simulink model "SIMULINK_anti-windup_anti-saturation"  (R2024b)
settings: Solver=ode45  StartTime=0.0  StopTime=1000  RelTol=1e-7  EnableMultiTasking=on
undefined symbols (not defined in the file): procede
settings Model: Creator=LiberT  LastModifiedBy=lordo
settings SolverCC: AlgebraicLoopSolver=TrustRegion
settings DataIOCC: LimitDataPoints=on  SaveFormat=Array  SignalLoggingSaveFormat=ModelDataLogs  ReturnWorkspaceOutputs=off
settings OptimizationCC: BlockReduction=off  BooleanDataType=off  ExpressionDepthLimit=2147483647  InitFltsAndDblsToZero=on  LifeSpan=inf
settings DebuggingCC: SaveWithParameterizedLinksMsg=none  UnderspecifiedInitializationDetection=Classic  MergeDetectMultiDrivingBlocksExec=none  SignalResolutionControl=TryResolveAllWithWarning  MultiTaskDSMMsg=warning  MultiTaskCondExecSysMsg=none  FcnCallInpInsideContextMsg=warning  UnconnectedInputMsg=warning  UnconnectedOutputMsg=warning  UnconnectedLineMsg=warning  StateNameClashWarn=warning  SFUnexpectedBacktrackingDiag=warning  SFNoUnconditionalDefaultTransitionDiag=warning  SFExecutionAtInitializationDiag=none  ArithmeticOperatorsInVariantConditions=warning
settings HardwareCC: ProdBitPerPointer=32  ProdBitPerSizeT=32  ProdBitPerPtrDiffT=32  ProdLargestAtomicFloat=None  ProdIntDivRoundTo=Undefined  ProdEndianess=Unspecified  ProdWordSize=32  ProdHWDeviceType=32-bit Generic  TargetUnknown=on
settings ModelReferenceCC: EnableRefExpFcnMdlSchedulingChecks=on  PropagateSignalLabelsOutOfModel=off
settings SFSimCC: SimUseLocalCustomCode=off  CustomCodeUndefinedFunction=UseInterfaceOnly
settings RTWCC: RTWUseLocalCustomCode=off  GPUComputeCapability=3.5
settings CodeAppCC: StateflowObjectComments=on
settings GRTTargetCC: TargetFcnLib=ansi_tfl_tmw.mat  TargetLangStandard=C89/C90 (ANSI)  ModelReferenceCompliant=off  CompOptLevelCompliant=off  CombineOutputUpdateFcns=off  MatFileLogging=off  GRTInterface=on
settings ConfigComp: CovMetricSettings=dw  CovSaveCumulativeToWorkspaceVar=on  CovSaveSingleToWorkspaceVar=on  CovExternalEMLEnable=off

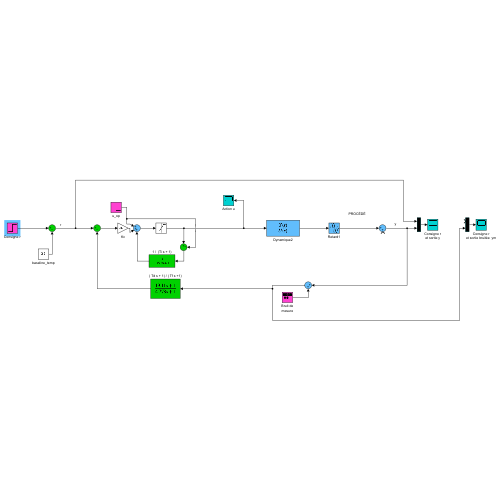
[thumbnail: Simulink's stored preview of the top-level diagram]
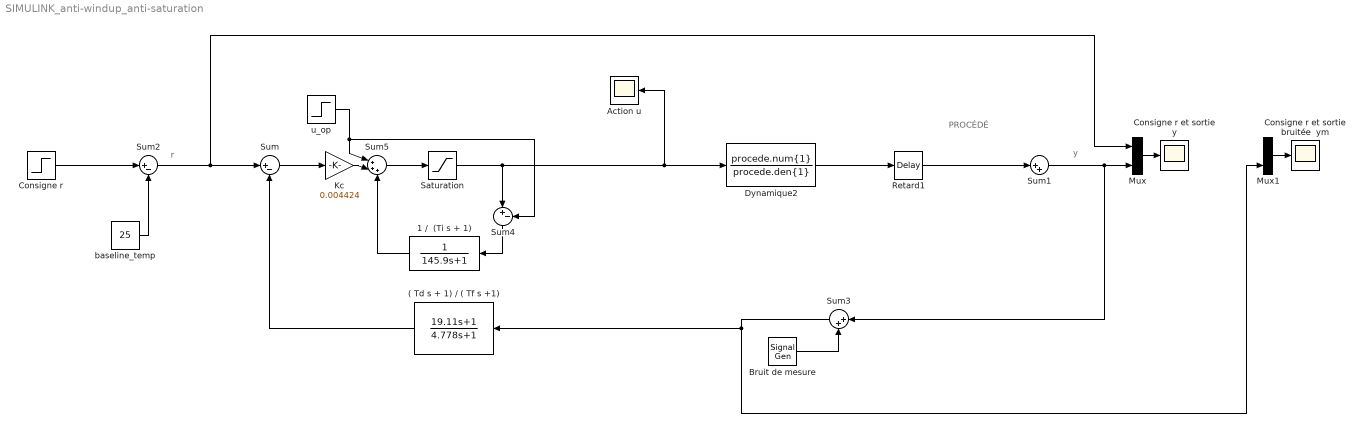
== system SIMULINK_anti-windup_anti-saturation ==
  note: PROCÉDÉ
  note: r
  note: y
  ( Td s + 1) / ( Tf s +1) : TransferFcn  Numerator=[19.11 1]  Denominator=[4.778 1]
  1 /  (Ti s + 1) : TransferFcn  Numerator=1  Denominator=[145.9 1]
  Action u : Scope
  Bruit de mesure : SignalGenerator  Amplitude=0  Units=rad/sec
  Consigne r : Step  Time=0  After=35  SampleTime=0
  Consigne r et sortie bruitée  ym : Scope
  Consigne r et sortie y : Scope
  Dynamique2 : TransferFcn  Numerator=procede.num{1}  Denominator=procede.den{1}
  Kc : Gain  Gain=0.004424
  Mux : Mux  Inputs=2
  Mux1 : Mux  Inputs=2
  Retard1 : TransportDelay  DelayTime=procede.InputDelay  BufferSize=5000
  Saturation : Saturate  UpperLimit=0.035  LowerLimit=-0.035
  Sum : Sum  Inputs=|+-  InputSameDT=on  SaturateOnIntegerOverflow=on  OutDataTypeStr=Inherit: Same as first input
  Sum1 : Sum  Inputs=|++  InputSameDT=on  SaturateOnIntegerOverflow=on  OutDataTypeStr=Inherit: Same as first input
  Sum2 : Sum  Inputs=|+-  InputSameDT=on  SaturateOnIntegerOverflow=on  OutDataTypeStr=Inherit: Same as first input
  Sum3 : Sum  Inputs=|++  InputSameDT=on  SaturateOnIntegerOverflow=on  OutDataTypeStr=Inherit: Same as first input
  Sum4 : Sum  Inputs=|+-  InputSameDT=on  SaturateOnIntegerOverflow=on  OutDataTypeStr=Inherit: Same as first input
  Sum5 : Sum  Inputs=|+++  InputSameDT=on  SaturateOnIntegerOverflow=on  OutDataTypeStr=Inherit: Same as first input
  baseline_temp : Constant  Value=25
  u_op : Step  Time=50  Before=0.005  After=0.000  SampleTime=0
  wires:
  Saturation/1 -> Dynamique2/1, Action u/1, Sum4/1
  Sum1/1 -> Mux/2, Sum3/1
  Mux/1 -> Consigne r et sortie y/1
  Sum3/1 -> Mux1/2, ( Td s + 1) / ( Tf s +1)/1
  Bruit de mesure/1 -> Sum3/2
  Mux1/1 -> Consigne r et sortie bruitée  ym/1
  Dynamique2/1 -> Retard1/1
  Retard1/1 -> Sum1/1
  u_op/1 -> Sum5/1, Sum4/2
  Sum4/1 -> 1 /  (Ti s + 1)/1
  1 /  (Ti s + 1)/1 -> Sum5/3
  Sum5/1 -> Saturation/1
  Kc/1 -> Sum5/2
  Sum/1 -> Kc/1
  ( Td s + 1) / ( Tf s +1)/1 -> Sum/2
  Sum2/1 -> Sum/1, Mux/1
  Consigne r/1 -> Sum2/1
  baseline_temp/1 -> Sum2/2
